simulink model "nmsRR"  (R2021a)
settings: Solver=ode15s  StartTime=0.0  StopTime=t  MaxStep=1e-2  RelTol=1e-2
StartFcn:
  | tic
StopFcn:
  | toc
  | 
  | 
  | %if GimbalLockFlag
  |  % fprintf(2, 'Almost reached Gimbal Lock of IMU. Simulation stopped.\n')
  | %end
  | 
  | %fprintf('Elapsed time: %4.2f sec (%4.2f%% realtime)\n', a, tout(end)/a*100)
undefined symbols (not defined in the file): Balance02, Balance13, BalanceTrunk, BasisStim, CompensateSwing, CompliantLeg, FlexAnkle, Ground, ICs, init_des_left, init_des_right, init_l_left, init_l_right, init_q_del, init_sensor_body, init_sensor_world, init_v_left, init_v_right, LateralControl, mParams, PreventKneeOverextension, StepDur, Target02, Target13, theta0, X, Y, Z
libraries: simulink_extras x133, nesl_utility x105, sm_lib x88, simulink x72, robotcorelib x5, dspinverses x5, dspswit3 x2, vrlib x2, robotmaniplib x1
(part 8 of 8)

== system nmsRR/Supraspinal Level/Subsystem/Compute Acceleration Profiles with Minimal Jerk Approach/Minimal jerk Hip Pitch4/Minimal Jerk Parameters [Movellan] ==
  x0 : Inport
  dx0 : Inport  Port=2
  ddx0 : Inport  Port=3
  xT : Inport  Port=4
  dxT : Inport  Port=5
  ddxT : Inport  Port=6
  T : Inport  Port=7
  Demux : Demux  Outputs=3
  Gain : Gain  Gain=0.5
  Gain1 : Gain  Gain=3
  Gain2 : Gain  Gain=6
  Gain3 : Gain  Gain=4
  Gain4 : Gain  Gain=12
  Gain5 : Gain  Gain=5
  Gain6 : Gain  Gain=20
  Matrix Multiply : Product  Multiplication=Matrix(*)
  Minus : Sum  Inputs=+---
  Minus1 : Sum  Inputs=+--
  Minus2 : Sum  Inputs=+-
  Mux : Mux  Inputs=6
  Mux{1..4} (4 alike) : Mux  Inputs=3
  Pseudoinverse : dspinverses/Pseudoinverse  wanterr=off  SimulateUsing=Code generation
      settings: SourceProductBaseCode=DS
  T{2..5} (4 alike) : Product  Inputs=**
  b : Concatenate  NumInputs=3  Mode=Multidimensional array  ConcatenateDimension=2
  multiply : Product  Inputs=**
  multiply1 : Product  Inputs=**
  multiply2 : Product  Inputs=**
  a : Outport
  wires:
  xT/1 -> Minus/1
  Minus1/1 -> Mux4/2
  T5/1 -> Mux3/1
  multiply1/1 -> Minus1/3
  Gain5/1 -> Mux3/2
  Demux/2 -> Mux/5
  dxT/1 -> Minus1/1
  Demux/3 -> Mux/6
  b/1 -> Pseudoinverse/1
  multiply2/1 -> Minus/3
  Minus2/1 -> Mux4/3
  Gain/1 -> multiply/1, Mux/3
  multiply/1 -> Minus/4
  ddxT/1 -> Minus2/1
  Gain4/1 -> Mux2/3
  Gain6/1 -> Mux3/3
  x0/1 -> Minus/2, Mux/1
  Mux1/1 -> b/1
  Matrix Multiply/1 -> Demux/1
  ddx0/1 -> Minus2/2, multiply1/1, Gain/1
  T2/1 -> Gain1/1, Gain4/1, T3/1, multiply/2
  Gain2/1 -> Mux1/3
  Mux4/1 -> Matrix Multiply/2
  T4/1 -> Mux2/1, Gain5/1, T5/1
  Minus/1 -> Mux4/1
  Pseudoinverse/1 -> Matrix Multiply/1
  Mux2/1 -> b/2
  Gain3/1 -> Mux2/2
  Mux3/1 -> b/3
  Gain1/1 -> Mux1/2
  T/1 -> multiply2/2, multiply1/2, Gain2/1, T5/2, T4/2, T3/2, T2/2, T2/1
  Demux/1 -> Mux/4
  Mux/1 -> a/1
  T3/1 -> Gain6/1, Gain3/1, Mux1/1, T4/1
  dx0/1 -> multiply2/1, Minus1/2, Mux/2

== system nmsRR/Supraspinal Level/Subsystem/Inverse Dynamics/Inverse Dynamics/Inverse Dynamics ==
  note: Inverse Dynamics: This block computes the 14 torques (joints(8), body rotation(3) and body translation(3)) needed to generate the desired joint accelerations compensating inertial, velocity depended and gravitational torques at the same time.
  Config : Inport
  JointVel : Inport  Port=2
  JointAccel : Inport  Port=3
  Constant2 : Constant  Value=zeros(6,15)
  Filtered Derrivative of torques : Subsystem  Commented=on
  Inverse Dynamics : robotmaniplib/Inverse Dynamics  RigidBodyTree=model_14dof  SimulateUsing=Code generation
      settings: SourceProductBaseCode=RO
  Select Body Joint Torques : Selector  InputPortWidth=14  IndexOptions=Index vector (dialog)  Indices=[7:14]  OutputSizes=1
  Desired Torques : Outport  VectorParamsAs1DForOutWhenUnconnected=off
  wires:
  Inverse Dynamics/1 -> Select Body Joint Torques/1
  Constant2/1 -> Inverse Dynamics/4
  Select Body Joint Torques/1 -> Desired Torques/1
  Config/1 -> Inverse Dynamics/1
  JointVel/1 -> Inverse Dynamics/2
  JointAccel/1 -> Inverse Dynamics/3

== system nmsRR/Supraspinal Level/Subsystem/torques --> forces/Moment Arm Matrix/Row 1 ==
  Constant : Constant  Value=mParams.muscles.HFL.r0
  Constant{1..18} (18 alike) : Constant  Value=0
  Constant19 : Constant  Value=-mParams.muscles.GLU.r0
  Constant20 : Constant  Value=-mParams.muscles.HAM.r0H
  Constant21 : Constant  Value=mParams.muscles.RF.r0H
  Mux2 : Mux  Inputs=22
  dl/theta1 : Outport
  wires:
  Constant3/1 -> Mux2/7
  Constant5/1 -> Mux2/8
  Constant8/1 -> Mux2/11
  Constant9/1 -> Mux2/13
  Constant4/1 -> Mux2/9
  Constant1/1 -> Mux2/2
  Constant2/1 -> Mux2/1
  Constant14/1 -> Mux2/17
  Constant7/1 -> Mux2/12
  Constant10/1 -> Mux2/15
  Constant6/1 -> Mux2/10
  Constant17/1 -> Mux2/22
  Constant15/1 -> Mux2/19
  Constant18/1 -> Mux2/21
  Constant11/1 -> Mux2/14
  Constant20/1 -> Mux2/5
  Constant12/1 -> Mux2/16
  Constant21/1 -> Mux2/6
  Constant19/1 -> Mux2/4
  Constant/1 -> Mux2/3
  Constant16/1 -> Mux2/20
  Constant13/1 -> Mux2/18
  Mux2/1 -> dl/theta1/1

== system nmsRR/Supraspinal Level/Subsystem/torques --> forces/Moment Arm Matrix/Row 2 ==
  Constant : Constant  Value=-mParams.muscles.HAB.r0
  Constant1 : Constant  Value=mParams.muscles.HAD.r0
  Constant{3..22} (20 alike) : Constant  Value=0
  Mux2 : Mux  Inputs=22
  dl/theta2 : Outport
  wires:
  Constant3/1 -> Mux2/7
  Constant5/1 -> Mux2/8
  Constant8/1 -> Mux2/11
  Constant9/1 -> Mux2/13
  Constant4/1 -> Mux2/9
  Constant1/1 -> Mux2/2
  Constant/1 -> Mux2/1
  Constant14/1 -> Mux2/17
  Constant7/1 -> Mux2/12
  Constant10/1 -> Mux2/15
  Constant6/1 -> Mux2/10
  Constant17/1 -> Mux2/22
  Constant15/1 -> Mux2/19
  Constant18/1 -> Mux2/21
  Constant11/1 -> Mux2/14
  Constant12/1 -> Mux2/16
  Constant16/1 -> Mux2/20
  Constant13/1 -> Mux2/18
  Mux2/1 -> dl/theta2/1
  Constant21/1 -> Mux2/4
  Constant20/1 -> Mux2/5
  Constant22/1 -> Mux2/6
  Constant19/1 -> Mux2/3

== system nmsRR/Supraspinal Level/Subsystem/torques --> forces/Moment Arm Matrix/Row 3 ==
  q(3) : Inport
  C(6,3) : Subsystem
  C(7,3) : Subsystem
  C(9,3) : Subsystem
  Constant : Constant  Value=mParams.muscles.BFSH.r0
  Constant{1..4,6..18} (17 alike) : Constant  Value=0
  Constant5 : Constant  Value=mParams.muscles.HAM.r0K
  Mux2 : Mux  Inputs=22
  dl/theta3 : Outport
  wires:
  C(7,3)/1(C(7,3)) -> Mux2/7
  Constant/1 -> Mux2/8
  Constant8/1 -> Mux2/11
  Constant9/1 -> Mux2/13
  C(9,3)/1(C(9,3)) -> Mux2/9
  Constant1/1 -> Mux2/2
  Constant2/1 -> Mux2/1
  Constant14/1 -> Mux2/17
  Constant7/1 -> Mux2/12
  Constant10/1 -> Mux2/15
  Constant6/1 -> Mux2/10
  Constant17/1 -> Mux2/22
  Constant15/1 -> Mux2/19
  Constant18/1 -> Mux2/21
  Constant11/1 -> Mux2/14
  Constant5/1 -> Mux2/5
  Constant12/1 -> Mux2/16
  Constant16/1 -> Mux2/20
  Constant13/1 -> Mux2/18
  Mux2/1 -> dl/theta3/1
  Constant4/1 -> Mux2/3
  Constant3/1 -> Mux2/4
  q(3)/1 -> C(7,3)/1(q(3)), C(9,3)/1(q(3)), C(6,3)/1(q(3))
  C(6,3)/1(C(6,3)) -> Mux2/6

== system nmsRR/Supraspinal Level/Subsystem/torques --> forces/Moment Arm Matrix/Row 4 ==
  q(4) : Inport
  C(10,4) : Subsystem
  C(11,4) : Subsystem
  C(9,4) : Subsystem
  Constant{1..3,5,7,9..22} (19 alike) : Constant  Value=0
  Mux2 : Mux  Inputs=22
  dl/theta4 : Outport
  wires:
  Constant3/1 -> Mux2/7
  Constant5/1 -> Mux2/8
  Constant9/1 -> Mux2/13
  Constant1/1 -> Mux2/2
  Constant2/1 -> Mux2/1
  Constant14/1 -> Mux2/17
  Constant7/1 -> Mux2/12
  Constant10/1 -> Mux2/15
  Constant17/1 -> Mux2/22
  Constant15/1 -> Mux2/19
  Constant18/1 -> Mux2/21
  Constant11/1 -> Mux2/14
  Constant12/1 -> Mux2/16
  Constant16/1 -> Mux2/20
  Constant13/1 -> Mux2/18
  Mux2/1 -> dl/theta4/1
  Constant19/1 -> Mux2/3
  Constant20/1 -> Mux2/5
  Constant21/1 -> Mux2/4
  Constant22/1 -> Mux2/6
  C(11,4)/1(C(11,4)) -> Mux2/11
  C(10,4)/1(C(10,4)) -> Mux2/10
  C(9,4)/1(C(9,4)) -> Mux2/9
  q(4)/1 -> C(11,4)/1(q(4)), C(10,4)/1(q(4)), C(9,4)/1(q(4))

== system nmsRR/Supraspinal Level/Subsystem/torques --> forces/Moment Arm Matrix/Row 5 ==
  Constant : Constant  Value=mParams.muscles.HFL.r0
  Constant{1..9,13,15..22} (18 alike) : Constant  Value=0
  Constant10 : Constant  Value=-mParams.muscles.GLU.r0
  Constant11 : Constant  Value=-mParams.muscles.HAM.r0H
  Constant12 : Constant  Value=mParams.muscles.RF.r0H
  Mux2 : Mux  Inputs=22
  dl/theta5 : Outport
  wires:
  Constant3/1 -> Mux2/7
  Constant5/1 -> Mux2/8
  Constant8/1 -> Mux2/11
  Constant9/1 -> Mux2/13
  Constant4/1 -> Mux2/9
  Constant1/1 -> Mux2/2
  Constant2/1 -> Mux2/1
  Constant12/1 -> Mux2/17
  Constant7/1 -> Mux2/12
  Constant6/1 -> Mux2/10
  Constant17/1 -> Mux2/22
  Constant15/1 -> Mux2/19
  Constant18/1 -> Mux2/21
  Constant16/1 -> Mux2/20
  Constant13/1 -> Mux2/18
  Mux2/1 -> dl/theta5/1
  Constant19/1 -> Mux2/3
  Constant21/1 -> Mux2/4
  Constant20/1 -> Mux2/5
  Constant22/1 -> Mux2/6
  Constant10/1 -> Mux2/15
  Constant11/1 -> Mux2/16
  Constant/1 -> Mux2/14

== system nmsRR/Supraspinal Level/Subsystem/torques --> forces/Moment Arm Matrix/Row 6 ==
  Constant : Constant  Value=-mParams.muscles.HAB.r0
  Constant{1..6,8,10..22} (20 alike) : Constant  Value=0
  Constant7 : Constant  Value=mParams.muscles.HAD.r0
  Mux2 : Mux  Inputs=22
  dl/theta6 : Outport
  wires:
  Constant3/1 -> Mux2/7
  Constant5/1 -> Mux2/8
  Constant8/1 -> Mux2/11
  Constant4/1 -> Mux2/9
  Constant1/1 -> Mux2/2
  Constant2/1 -> Mux2/1
  Constant14/1 -> Mux2/17
  Constant10/1 -> Mux2/15
  Constant6/1 -> Mux2/10
  Constant17/1 -> Mux2/22
  Constant15/1 -> Mux2/19
  Constant18/1 -> Mux2/21
  Constant11/1 -> Mux2/14
  Constant12/1 -> Mux2/16
  Constant16/1 -> Mux2/20
  Constant13/1 -> Mux2/18
  Mux2/1 -> dl/theta6/1
  Constant20/1 -> Mux2/5
  Constant21/1 -> Mux2/4
  Constant19/1 -> Mux2/3
  Constant22/1 -> Mux2/6
  Constant/1 -> Mux2/12
  Constant7/1 -> Mux2/13

== system nmsRR/Supraspinal Level/Subsystem/torques --> forces/Moment Arm Matrix/Row 7 ==
  q(7) : Inport
  C(17,7) : Subsystem
  C(18,7) : Subsystem
  C(20,7) : Subsystem
  Constant : Constant  Value=mParams.muscles.BFSH.r0
  Constant{1..11,17..22} (17 alike) : Constant  Value=0
  Constant13 : Constant  Value=mParams.muscles.HAM.r0K
  Mux2 : Mux  Inputs=22
  dl/theta7 : Outport
  wires:
  Constant3/1 -> Mux2/7
  Constant5/1 -> Mux2/8
  Constant8/1 -> Mux2/11
  Constant9/1 -> Mux2/13
  Constant4/1 -> Mux2/9
  Constant1/1 -> Mux2/2
  Constant2/1 -> Mux2/1
  Constant7/1 -> Mux2/12
  Constant10/1 -> Mux2/15
  Constant6/1 -> Mux2/10
  Constant17/1 -> Mux2/22
  Constant18/1 -> Mux2/21
  Constant11/1 -> Mux2/14
  C(20,7)/1(C(20,7)) -> Mux2/20
  Mux2/1 -> dl/theta7/1
  Constant20/1 -> Mux2/5
  Constant21/1 -> Mux2/4
  Constant19/1 -> Mux2/3
  Constant22/1 -> Mux2/6
  Constant13/1 -> Mux2/16
  C(18,7)/1(C(18,7)) -> Mux2/18
  C(17,7)/1(C(17,7)) -> Mux2/17
  Constant/1 -> Mux2/19
  q(7)/1 -> C(18,7)/1(q(7)), C(20,7)/1(q(7)), C(17,7)/1(q(7))

== system nmsRR/Supraspinal Level/Subsystem/torques --> forces/Moment Arm Matrix/Row 8 ==
  q(8) : Inport
  C(10,4) : Subsystem
  C(11,4) : Subsystem
  C(9,4) : Subsystem
  Constant{1..15,19..22} (19 alike) : Constant  Value=0
  Mux2 : Mux  Inputs=22
  dl/theta8 : Outport
  wires:
  Constant3/1 -> Mux2/7
  Constant5/1 -> Mux2/8
  Constant8/1 -> Mux2/11
  Constant9/1 -> Mux2/13
  Constant4/1 -> Mux2/9
  Constant1/1 -> Mux2/2
  Constant2/1 -> Mux2/1
  Constant14/1 -> Mux2/17
  Constant7/1 -> Mux2/12
  Constant10/1 -> Mux2/15
  Constant6/1 -> Mux2/10
  C(11,4)/1(C(22,8)) -> Mux2/22
  Constant15/1 -> Mux2/19
  Constant11/1 -> Mux2/14
  Constant12/1 -> Mux2/16
  Constant13/1 -> Mux2/18
  Mux2/1 -> dl/theta8/1
  Constant19/1 -> Mux2/3
  Constant21/1 -> Mux2/4
  Constant20/1 -> Mux2/5
  Constant22/1 -> Mux2/6
  C(10,4)/1(C(21,8)) -> Mux2/21
  q(8)/1 -> C(11,4)/1(q(8)), C(10,4)/1(q(8)), C(9,4)/1(q(8))
  C(9,4)/1(C(20,8)) -> Mux2/20

== system nmsRR/Supraspinal Level/Subsystem/torques --> forces/Subsystem1/F from T ==
  T : Inport
  Matrix Multiply : Product  Multiplication=Matrix(*)
  F : Outport
  wires:
  T/1 -> Matrix Multiply/2
  Matrix Multiply/1 -> F/1
  [C_transpose] -> Matrix Multiply/1

== system nmsRR/Supraspinal Level/Subsystem/torques --> forces/Subsystem1/T from F ==
  F : Inport
  Matrix Multiply : Product  Multiplication=Matrix(*)
  Transpose : Math  Operator=transpose  SaturateOnIntegerOverflow=on
  T : Outport
  wires:
  Matrix Multiply/1 -> T/1
  F/1 -> Matrix Multiply/2
  Transpose/1 -> Matrix Multiply/1
  [C] -> Transpose/1

== system nmsRR/Supraspinal Level/Subsystem/torques --> forces/Subsystem1/separate Force ==
  Force : Inport
  Constant4 : Constant  Value=zeros(22,1)
  Max2 : MinMax  Function=max  Inputs=2  OutDataTypeStr=double  ZeroCross=off
  Max3 : MinMax  Inputs=2  OutDataTypeStr=double  ZeroCross=off
  Positive Part : Outport
  Negative Part : Outport  Port=2
  wires:
  Max3/1 -> Negative Part/1
  Max2/1 -> Positive Part/1
  Force/1 -> Max3/1, Max2/1
  Constant4/1 -> Max3/2, Max2/2

== system nmsRR/Supraspinal Level/Subsystem/torques --> forces/Subsystem12/F from T ==
  T : Inport
  Matrix Multiply : Product  Multiplication=Matrix(*)
  F : Outport
  wires:
  T/1 -> Matrix Multiply/2
  Matrix Multiply/1 -> F/1
  [C_transpose] -> Matrix Multiply/1

== system nmsRR/Supraspinal Level/Subsystem/torques --> forces/Subsystem12/T from F ==
  F : Inport
  Matrix Multiply : Product  Multiplication=Matrix(*)
  Transpose : Math  Operator=transpose  SaturateOnIntegerOverflow=on
  T : Outport
  wires:
  Matrix Multiply/1 -> T/1
  F/1 -> Matrix Multiply/2
  Transpose/1 -> Matrix Multiply/1
  [C] -> Transpose/1

== system nmsRR/Supraspinal Level/Subsystem/torques --> forces/Subsystem12/separate Force ==
  Force : Inport
  Constant4 : Constant  Value=zeros(22,1)
  Max2 : MinMax  Function=max  Inputs=2  OutDataTypeStr=double  ZeroCross=off
  Max3 : MinMax  Inputs=2  OutDataTypeStr=double  ZeroCross=off
  Positive Part : Outport
  Negative Part : Outport  Port=2
  wires:
  Max3/1 -> Negative Part/1
  Max2/1 -> Positive Part/1
  Force/1 -> Max3/1, Max2/1
  Constant4/1 -> Max3/2, Max2/2

== system nmsRR/Supraspinal Level/Subsystem/torques --> forces/Subsystem2/F from T ==
  T : Inport
  Matrix Multiply : Product  Multiplication=Matrix(*)
  F : Outport
  wires:
  T/1 -> Matrix Multiply/2
  Matrix Multiply/1 -> F/1
  [C_transpose] -> Matrix Multiply/1

== system nmsRR/Supraspinal Level/Subsystem/torques --> forces/Subsystem2/T from F ==
  F : Inport
  Matrix Multiply : Product  Multiplication=Matrix(*)
  Transpose : Math  Operator=transpose  SaturateOnIntegerOverflow=on
  T : Outport
  wires:
  Matrix Multiply/1 -> T/1
  F/1 -> Matrix Multiply/2
  Transpose/1 -> Matrix Multiply/1
  [C] -> Transpose/1

== system nmsRR/Supraspinal Level/Subsystem/torques --> forces/Subsystem2/separate Force ==
  Force : Inport
  Constant4 : Constant  Value=zeros(22,1)
  Max2 : MinMax  Function=max  Inputs=2  OutDataTypeStr=double  ZeroCross=off
  Max3 : MinMax  Inputs=2  OutDataTypeStr=double  ZeroCross=off
  Positive Part : Outport
  Negative Part : Outport  Port=2
  wires:
  Max3/1 -> Negative Part/1
  Max2/1 -> Positive Part/1
  Force/1 -> Max3/1, Max2/1
  Constant4/1 -> Max3/2, Max2/2

== system nmsRR/Supraspinal Level/Subsystem/torques --> forces/Subsystem3/F from T ==
  T : Inport
  Matrix Multiply : Product  Multiplication=Matrix(*)
  F : Outport
  wires:
  T/1 -> Matrix Multiply/2
  Matrix Multiply/1 -> F/1
  [C_transpose] -> Matrix Multiply/1

== system nmsRR/Supraspinal Level/Subsystem/torques --> forces/Subsystem3/T from F ==
  F : Inport
  Matrix Multiply : Product  Multiplication=Matrix(*)
  Transpose : Math  Operator=transpose  SaturateOnIntegerOverflow=on
  T : Outport
  wires:
  Matrix Multiply/1 -> T/1
  F/1 -> Matrix Multiply/2
  Transpose/1 -> Matrix Multiply/1
  [C] -> Transpose/1

== system nmsRR/Supraspinal Level/Subsystem/torques --> forces/Subsystem3/separate Force ==
  Force : Inport
  Constant4 : Constant  Value=zeros(22,1)
  Max2 : MinMax  Function=max  Inputs=2  OutDataTypeStr=double  ZeroCross=off
  Max3 : MinMax  Inputs=2  OutDataTypeStr=double  ZeroCross=off
  Positive Part : Outport
  Negative Part : Outport  Port=2
  wires:
  Max3/1 -> Negative Part/1
  Max2/1 -> Positive Part/1
  Force/1 -> Max3/1, Max2/1
  Constant4/1 -> Max3/2, Max2/2

== system nmsRR/Supraspinal Level/Subsystem/torques --> forces/Subsystem4/F from T ==
  T : Inport
  Matrix Multiply : Product  Multiplication=Matrix(*)
  F : Outport
  wires:
  T/1 -> Matrix Multiply/2
  Matrix Multiply/1 -> F/1
  [C_transpose] -> Matrix Multiply/1

== system nmsRR/Supraspinal Level/Subsystem/torques --> forces/Subsystem4/T from F ==
  F : Inport
  Matrix Multiply : Product  Multiplication=Matrix(*)
  Transpose : Math  Operator=transpose  SaturateOnIntegerOverflow=on
  T : Outport
  wires:
  Matrix Multiply/1 -> T/1
  F/1 -> Matrix Multiply/2
  Transpose/1 -> Matrix Multiply/1
  [C] -> Transpose/1

== system nmsRR/Supraspinal Level/Subsystem/torques --> forces/Subsystem4/separate Force ==
  Force : Inport
  Constant4 : Constant  Value=zeros(22,1)
  Max2 : MinMax  Function=max  Inputs=2  OutDataTypeStr=double  ZeroCross=off
  Max3 : MinMax  Inputs=2  OutDataTypeStr=double  ZeroCross=off
  Positive Part : Outport
  Negative Part : Outport  Port=2
  wires:
  Max3/1 -> Negative Part/1
  Max2/1 -> Positive Part/1
  Force/1 -> Max3/1, Max2/1
  Constant4/1 -> Max3/2, Max2/2

== system nmsRR/Supraspinal Level/Subsystem/Inverse Dynamics/Inverse Dynamics/Inverse Dynamics/Filtered Derrivative of torques ==
  " [1x8]" : Inport
  Demux : Demux  Outputs=8
  Filtered Derivative{1..8} (8 alike) : TransferFcn  Numerator=[1 0]  Denominator=[0.001 1]
  Mux : Mux  Inputs=8
  "[1x8]" : Outport  VectorParamsAs1DForOutWhenUnconnected=off
  wires:
  Mux/1 -> "[1x8]"/1
  " [1x8]"/1 -> Demux/1
  Filtered Derivative5/1 -> Mux/1  "Filt. Der. 1"
  Filtered Derivative6/1 -> Mux/2  "Filt. Der. 1"
  Filtered Derivative7/1 -> Mux/3  "Filt. Der. 1"
  Filtered Derivative8/1 -> Mux/4  "Filt. Der. 1"
  Filtered Derivative1/1 -> Mux/5  "Filt. Der. 1"
  Filtered Derivative2/1 -> Mux/6  "Filt. Der. 1"
  Filtered Derivative3/1 -> Mux/7  "Filt. Der. 1"
  Filtered Derivative4/1 -> Mux/8  "Filt. Der. 1"
  Demux/1 -> Filtered Derivative5/1
  Demux/2 -> Filtered Derivative6/1
  Demux/3 -> Filtered Derivative7/1
  Demux/4 -> Filtered Derivative8/1
  Demux/5 -> Filtered Derivative1/1
  Demux/6 -> Filtered Derivative2/1
  Demux/7 -> Filtered Derivative3/1
  Demux/8 -> Filtered Derivative4/1

== system nmsRR/Supraspinal Level/Subsystem/torques --> forces/Moment Arm Matrix/Row 3/C(6,3) ==
  q(3) : Inport
  Constant20 : Constant  Value=mParams.muscles.RF.qMxK
  Constant21 : Constant  Value=mParams.muscles.RF.c0K
  Constant5 : Constant  Value=mParams.muscles.RF.rMxK
  Gain : Gain  Gain=-1
  Minus : Sum  Inputs=+-
  Minus1 : Sum  Inputs=+-
  Product : Product
  Square : Math  Operator=square  SaturateOnIntegerOverflow=on
  C(6,3) : Outport
  wires:
  Constant21/1 -> Product/1
  Constant20/1 -> Minus1/2
  Constant5/1 -> Minus/1
  q(3)/1 -> Minus1/1
  Minus/1 -> Gain/1
  Product/1 -> Minus/2
  Gain/1 -> C(6,3)/1
  Minus1/1 -> Square/1
  Square/1 -> Product/2

== system nmsRR/Supraspinal Level/Subsystem/torques --> forces/Moment Arm Matrix/Row 3/C(7,3) ==
  q(3) : Inport
  Constant1 : Constant  Value=-mParams.muscles.VAS.rMx
  Constant2 : Constant  Value=mParams.muscles.VAS.c0
  Constant20 : Constant  Value=mParams.muscles.VAS.qMx
  Minus1 : Sum  Inputs=+-
  Minus2 : Sum
  Product1 : Product
  Square1 : Math  Operator=square  SaturateOnIntegerOverflow=on
  C(7,3) : Outport
  wires:
  Constant20/1 -> Minus1/2
  q(3)/1 -> Minus1/1
  Constant1/1 -> Minus2/1
  Product1/1 -> Minus2/2
  Constant2/1 -> Product1/1
  Minus1/1 -> Square1/1
  Minus2/1 -> C(7,3)/1
  Square1/1 -> Product1/2

== system nmsRR/Supraspinal Level/Subsystem/torques --> forces/Moment Arm Matrix/Row 3/C(9,3) ==
  q(3) : Inport
  Constant20 : Constant  Value=mParams.muscles.GAS.qMxK
  Constant21 : Constant  Value=mParams.muscles.GAS.c0K
  Constant5 : Constant  Value=mParams.muscles.GAS.rMxK
  Minus : Sum  Inputs=+-
  Minus1 : Sum  Inputs=+-
  Product : Product
  Square : Math  Operator=square  SaturateOnIntegerOverflow=on
  C(9,3) : Outport
  wires:
  Constant21/1 -> Product/1
  Constant20/1 -> Minus1/2
  Constant5/1 -> Minus/1
  q(3)/1 -> Minus1/1
  Product/1 -> Minus/2
  Minus/1 -> C(9,3)/1
  Minus1/1 -> Square/1
  Square/1 -> Product/2

== system nmsRR/Supraspinal Level/Subsystem/torques --> forces/Moment Arm Matrix/Row 4/C(10,4) ==
  q(4) : Inport
  Constant1 : Constant  Value=-mParams.muscles.SOL.rMx
  Constant2 : Constant  Value=mParams.muscles.SOL.c0
  Constant20 : Constant  Value=mParams.muscles.SOL.qMx
  Minus1 : Sum  Inputs=+-
  Minus2 : Sum
  Product1 : Product
  Square1 : Math  Operator=square  SaturateOnIntegerOverflow=on
  C(10,4) : Outport
  wires:
  Constant20/1 -> Minus1/2
  q(4)/1 -> Minus1/1
  Constant1/1 -> Minus2/1
  Product1/1 -> Minus2/2
  Constant2/1 -> Product1/1
  Minus1/1 -> Square1/1
  Minus2/1 -> C(10,4)/1
  Square1/1 -> Product1/2

== system nmsRR/Supraspinal Level/Subsystem/torques --> forces/Moment Arm Matrix/Row 4/C(11,4) ==
  q(4) : Inport
  Constant1 : Constant  Value=mParams.muscles.TA.rMx
  Constant2 : Constant  Value=mParams.muscles.TA.c0
  Constant20 : Constant  Value=mParams.muscles.TA.qMx
  Minus1 : Sum  Inputs=+-
  Minus2 : Sum  Inputs=+-
  Product1 : Product
  Square1 : Math  Operator=square  SaturateOnIntegerOverflow=on
  C(11,4) : Outport
  wires:
  Constant20/1 -> Minus1/2
  q(4)/1 -> Minus1/1
  Constant1/1 -> Minus2/1
  Product1/1 -> Minus2/2
  Constant2/1 -> Product1/1
  Minus1/1 -> Square1/1
  Minus2/1 -> C(11,4)/1
  Square1/1 -> Product1/2

== system nmsRR/Supraspinal Level/Subsystem/torques --> forces/Moment Arm Matrix/Row 4/C(9,4) ==
  q(4) : Inport
  Constant20 : Constant  Value=mParams.muscles.GAS.qMxA
  Constant21 : Constant  Value=mParams.muscles.GAS.c0A
  Constant5 : Constant  Value=mParams.muscles.GAS.rMxA
  Gain : Gain  Gain=-1
  Minus : Sum  Inputs=+-
  Minus1 : Sum  Inputs=+-
  Product : Product
  Square : Math  Operator=square  SaturateOnIntegerOverflow=on
  C(9,4) : Outport
  wires:
  Constant21/1 -> Product/1
  Constant20/1 -> Minus1/2
  Constant5/1 -> Minus/1
  q(4)/1 -> Minus1/1
  Product/1 -> Minus/2
  Minus/1 -> Gain/1
  Minus1/1 -> Square/1
  Square/1 -> Product/2
  Gain/1 -> C(9,4)/1

== system nmsRR/Supraspinal Level/Subsystem/torques --> forces/Moment Arm Matrix/Row 7/C(17,7) ==
  q(7) : Inport
  Constant20 : Constant  Value=mParams.muscles.RF.qMxK
  Constant21 : Constant  Value=mParams.muscles.RF.c0K
  Constant5 : Constant  Value=mParams.muscles.RF.rMxK
  Gain : Gain  Gain=-1
  Minus : Sum  Inputs=+-
  Minus1 : Sum  Inputs=+-
  Product : Product
  Square : Math  Operator=square  SaturateOnIntegerOverflow=on
  C(17,7) : Outport
  wires:
  Constant21/1 -> Product/1
  Constant20/1 -> Minus1/2
  Constant5/1 -> Minus/1
  q(7)/1 -> Minus1/1
  Minus/1 -> Gain/1
  Product/1 -> Minus/2
  Gain/1 -> C(17,7)/1
  Minus1/1 -> Square/1
  Square/1 -> Product/2

== system nmsRR/Supraspinal Level/Subsystem/torques --> forces/Moment Arm Matrix/Row 7/C(18,7) ==
  q(7) : Inport
  Constant1 : Constant  Value=-mParams.muscles.VAS.rMx
  Constant2 : Constant  Value=mParams.muscles.VAS.c0
  Constant20 : Constant  Value=mParams.muscles.VAS.qMx
  Minus1 : Sum  Inputs=+-
  Minus2 : Sum
  Product1 : Product
  Square1 : Math  Operator=square  SaturateOnIntegerOverflow=on
  C(18,7) : Outport
  wires:
  Constant20/1 -> Minus1/2
  q(7)/1 -> Minus1/1
  Constant1/1 -> Minus2/1
  Product1/1 -> Minus2/2
  Constant2/1 -> Product1/1
  Minus1/1 -> Square1/1
  Minus2/1 -> C(18,7)/1
  Square1/1 -> Product1/2

== system nmsRR/Supraspinal Level/Subsystem/torques --> forces/Moment Arm Matrix/Row 7/C(20,7) ==
  q(7) : Inport
  Constant20 : Constant  Value=mParams.muscles.GAS.qMxK
  Constant21 : Constant  Value=mParams.muscles.GAS.c0K
  Constant5 : Constant  Value=mParams.muscles.GAS.rMxK
  Minus : Sum  Inputs=+-
  Minus1 : Sum  Inputs=+-
  Product : Product
  Square : Math  Operator=square  SaturateOnIntegerOverflow=on
  C(20,7) : Outport
  wires:
  Constant21/1 -> Product/1
  Constant20/1 -> Minus1/2
  Constant5/1 -> Minus/1
  q(7)/1 -> Minus1/1
  Product/1 -> Minus/2
  Minus/1 -> C(20,7)/1
  Minus1/1 -> Square/1
  Square/1 -> Product/2

== system nmsRR/Supraspinal Level/Subsystem/torques --> forces/Moment Arm Matrix/Row 8/C(10,4) ==
  q(8) : Inport
  Constant1 : Constant  Value=-mParams.muscles.SOL.rMx
  Constant2 : Constant  Value=mParams.muscles.SOL.c0
  Constant20 : Constant  Value=mParams.muscles.SOL.qMx
  Minus1 : Sum  Inputs=+-
  Minus2 : Sum
  Product1 : Product
  Square1 : Math  Operator=square  SaturateOnIntegerOverflow=on
  C(21,8) : Outport
  wires:
  Constant20/1 -> Minus1/2
  q(8)/1 -> Minus1/1
  Constant1/1 -> Minus2/1
  Product1/1 -> Minus2/2
  Constant2/1 -> Product1/1
  Minus1/1 -> Square1/1
  Minus2/1 -> C(21,8)/1
  Square1/1 -> Product1/2

== system nmsRR/Supraspinal Level/Subsystem/torques --> forces/Moment Arm Matrix/Row 8/C(11,4) ==
  q(8) : Inport
  Constant1 : Constant  Value=mParams.muscles.TA.rMx
  Constant2 : Constant  Value=mParams.muscles.TA.c0
  Constant20 : Constant  Value=mParams.muscles.TA.qMx
  Minus1 : Sum  Inputs=+-
  Minus2 : Sum  Inputs=+-
  Product1 : Product
  Square1 : Math  Operator=square  SaturateOnIntegerOverflow=on
  C(22,8) : Outport
  wires:
  Constant20/1 -> Minus1/2
  q(8)/1 -> Minus1/1
  Constant1/1 -> Minus2/1
  Product1/1 -> Minus2/2
  Constant2/1 -> Product1/1
  Minus1/1 -> Square1/1
  Minus2/1 -> C(22,8)/1
  Square1/1 -> Product1/2

== system nmsRR/Supraspinal Level/Subsystem/torques --> forces/Moment Arm Matrix/Row 8/C(9,4) ==
  q(8) : Inport
  Constant20 : Constant  Value=mParams.muscles.GAS.qMxA
  Constant21 : Constant  Value=mParams.muscles.GAS.c0A
  Constant5 : Constant  Value=mParams.muscles.GAS.rMxA
  Gain : Gain  Gain=-1
  Minus : Sum  Inputs=+-
  Minus1 : Sum  Inputs=+-
  Product : Product
  Square : Math  Operator=square  SaturateOnIntegerOverflow=on
  C(20,8) : Outport
  wires:
  Constant21/1 -> Product/1
  Constant20/1 -> Minus1/2
  Constant5/1 -> Minus/1
  q(8)/1 -> Minus1/1
  Product/1 -> Minus/2
  Minus/1 -> Gain/1
  Minus1/1 -> Square/1
  Square/1 -> Product/2
  Gain/1 -> C(20,8)/1

== stateflow chart nmsRR/Supraspinal Level/Finite State Machine/Chart ==
  settings: executeAtInitialization=1
  state State0
    entry:
    state0=1;
    state1=0;
    state2=0;
    state3=0;
  state State1
    entry:
    state0=0;
    state1=1;
    state2=0;
    state3=0;
  state State3
    entry:
    state0=0;
    state1=0;
    state2=0;
    state3=1;
  state State2
    entry:
    state0=0;
    state1=0;
    state2=1;
    state3=0;
  (default) -> State0
  State0 -> State1 : after(dt,sec)
  State3 -> State0 : [contact_left]
  State1 -> State2 : [contact_right]
  State2 -> State3 : after(dt,sec)
  data: state0 output; state1 output; state2 output; state3 output; dt input; contact_left input; contact_right input
